simulink library "vmc"  (R2021b)
settings: Solver=VariableStepAuto  StartTime=0.0  StopTime=10.0  RelTol=1e-3
undefined symbols (not defined in the file or in its folder): AVMC_ACCDeltaTqIGain_X_kph, AVMC_ACCDeltaTqIGain_Y_mps2, AVMC_ACCDeltaTqPGain_X_kph, AVMC_ACCDeltaTqPGain_Y_kph, AVMC_ACCLongSteadyCtrl_X_kph, AVMC_AggressJerkPCT4AT_X_kph, AVMC_AggressJerkPCT_X_kph, AVMC_AggressLimitPCT4AT_X_kph, AVMC_AggressLimitPCT_X_kph, AVMC_CCLongSteadyCtrl_X_kph, AVMC_DISCDeltaTqIGain_X_kph, AVMC_DISCDeltaTqIGain_Y_mps2, AVMC_DISCDeltaTqPGain_X_kph, AVMC_DISCDeltaTqPGain_Y_kph, AVMC_DISCTrunAccJerk_X_s, AVMC_DISCTrunAccLimit_X_s, AVMC_ESCRegenOut_X_kph, AVMC_ESCRegenOut_Y_Deg, AVMC_ESCRegenOutEnSpd_X_Deg, AVMC_ISOAccLimit_X_mps, AVMC_ISODecLimit_X_mps, AVMC_ISOJerk_X_mps, AVMC_LatESCRegenOut_X_kph, AVMC_LatESCRegenOut_Y_Deg, AVMC_LongAccDeadZone_X_kph, AVMC_LongAccFiltTsforP2_X_Gps, AVMC_MCPresBaseTq_X_bar, AVMC_MSALongSteadyCtrl_X_kph, AVMC_MSAPedalOvrd2_X_kph, AVMC_MSAPedalOvrd_X_kph, AVMC_MSASpdBand_X_kph, AVMC_MSATqDownEndTq_X_kph, AVMC_MSATqDownTime_X_kph, AVMC_RDCDetectTime_X_kph, AVMC_RDCDetectTime_Y_pct, AVMC_RDCEnSlideRate_X_Deg, AVMC_RearWhlTqRatio_X_Nm, AVMC_RearWhlTqRatio_Y_gps, AVMC_RearWhlTqSlipGain_X_rat, AVMC_RearWhlTqSlipGain_Y_kph, AVMC_SoftJerkPCT_X_kph, AVMC_SoftLimitPCT_X_kph, AVMC_StESCYaw_X_kph, AVMC_StESCYaw_Y_Deg, AVMC_StESCYawCom_X_kph, AVMC_StESCYawCom_Y_Gps, AVMC_TMSpdBaseTq_X_rpm, AVMC_VehHoldBDecMap_X_kph, AVMC_VehHoldDecCtrlTime_X_kph, AVMC_VehHoldMCPPass_X_deg, C_TASK_10MS_S, C_TASK_5MS_S, DEG2RAD, Discrete, ENUM_ACCAVAIL_AVAILABLE, ENUM_ACCCTRLALLOW_ALLOW, ENUM_ADASACCSTA_ACTIVE, ENUM_ADASACCSTA_OVERRIDE, ENUM_ADASACCSTA_SHUTOFF, ENUM_ADASAEBREQ_NOREQUEST ... (+361)
libraries: hcu_lib x63, simulink x60, simulink_extras x3, ctrlSharedLib x3, $bdroot x2
(part 7 of 15)

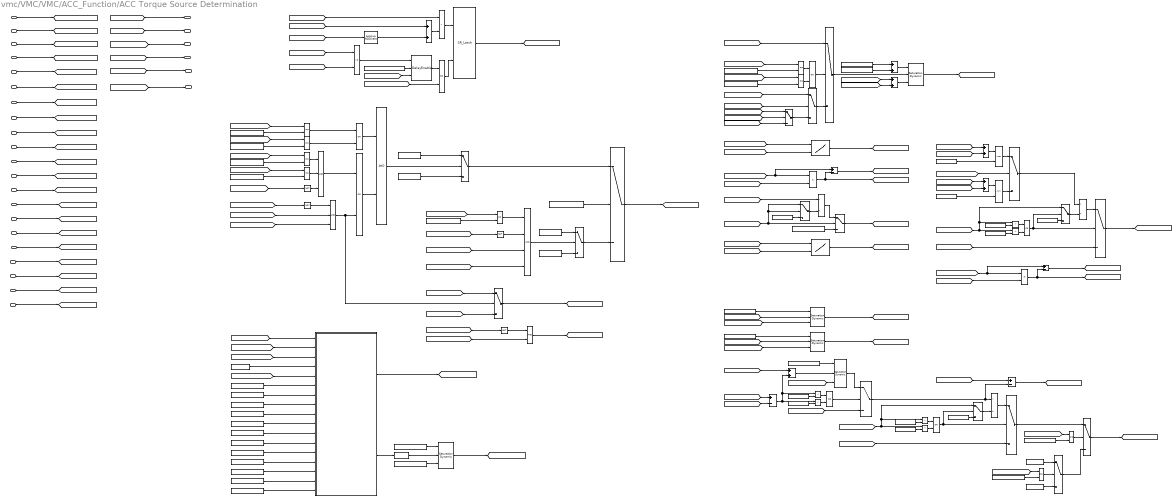
== system vmc/VMC/VMC/ACC_Function/ACC Torque Source Determination ==
  note: TRUE
  VTQD_DriverWhlTqDem_Nm : Inport
  VVMC_ADASWhlTqCal_Nm : Inport  Port=2
  VVMC_FeatArbitrFinal_enum : Inport  Port=3
  VTQD_LowIdleAccPedal_flg : Inport  Port=4
  VINP_ACCObjDist_m : Inport  Port=5
  VINP_TimeGapLevel_enum : Inport  Port=6
  VVMC_FeatArbitrSta_enum : Inport  Port=7
  VINP_RegenMode_enum : Inport  Port=8
  VVMC_ADASActive_flg : Inport  Port=9
  task_time_s : Inport  Port=10
  VINP_LongAccel_Gps : Inport  Port=11
  VINP_VehSpeed_kph : Inport  Port=12
  VVMC_FrRrSlipSpd_kph : Inport  Port=13
  VVMC_CruzWhlTqReq_Nm : Inport  Port=14
  VVMC_CruzActive_flg : Inport  Port=15
  VVMC_MSAWhlTqReq_Nm : Inport  Port=16
  VVMC_MSAActive_flg : Inport  Port=17
  VTQD_RrEDUAvailBrkRgnTq_Nm : Inport  Port=18
  VTQD_FrEDUAvailBrkRgnTq_Nm : Inport  Port=19
  VPMM_DrivetrainSelect_enum : Inport  Port=20
  VINP_ACCObjRelSpd_mps : Inport  Port=21
  AND : Logic  AllPortsSameDT=off  OutDataTypeStr=boolean
  AND1 : Logic  Inputs=4  AllPortsSameDT=off  OutDataTypeStr=boolean
  AND2 : Logic  Operator=OR  AllPortsSameDT=off  OutDataTypeStr=boolean
  AND3 : Logic  Operator=OR  AllPortsSameDT=off  OutDataTypeStr=boolean
  AND4 : Logic  Operator=OR  AllPortsSameDT=off  OutDataTypeStr=boolean
  Add{,2..3,9..11} (6 alike) : Sum
  Add{1,4..6} (4 alike) : Sum  Inputs=+-
  Cast To Single : DataTypeConversion  OutDataTypeStr=single
  Constant : Constant  Value=KVMC_ACCPedalOvrdSWC_flg
  Constant1 : Constant  Value=FALSE
  Constant10 : Constant  Value=ENUM_TIMEGAPLEVEL_LEVEL1
  Constant11 : Constant  Value=ENUM_TIMEGAPLEVEL_LEVEL2
  Constant12 : Constant  Value=ENUM_TIMEGAPLEVEL_LEVEL3
  Constant13 : Constant  Value=ENUM_TIMEGAPLEVEL_LEVEL4
  Constant14 : Constant  Value=KVMC_TimeGapBandLv2_s
  Constant15 : Constant  Value=KVMC_TimeGapBandLv3_s
  Constant16 : Constant  Value=KVMC_TimeGapBandLv4_s
  Constant17 : Constant  Value=TRUE
  Constant18 : Constant  Value=FALSE
  Constant{19,24..26,39,41..46,48} (12 alike) : Constant  Value=ZERO_FLOAT
  Constant2 : Constant  Value=ENUM_FEATARBITRSTA_DISC
  Constant20 : Constant  Value=FALSE
  Constant21 : Constant  Value=ENUM_FEATARBITRSTA_ACC
  Constant22 : Constant  Value=TRUE
  Constant23 : Constant  Value=KVMC_ACCPedalOvrdRestTime_s
  Constant{27..28,37,40} (4 alike) : Constant  Value=ONE_FLOAT
  Constant29 : Constant  Value=ENUM_FEATARBITRSTA_ACC
  Constant3 : Constant  Value=TRUE
  Constant30 : Constant  Value=ENUM_FEATARBITRSTA_DISC
  Constant31 : Constant  Value=KTQD_RrUppTheldTrq_Nm
  Constant32 : Constant  Value=ENUM_DRIVETRAIN_AWD  VectorParams1D=off  SampleTime=-1
  Constant33 : Constant  Value=KTQD_RrUppTheldTrq_Nm
  Constant34 : Constant  Value=KTQD_RrUppTheldTrq_Nm
  Constant35 : Constant  Value=KTQD_FrUppTheldTrq_Nm
  Constant36 : Constant  Value=KTQD_FrUppTheldTrq_Nm
  Constant38 : Constant  Value=ENUM_DRIVETRAIN_RWD  VectorParams1D=off  SampleTime=-1
  Constant4 : Constant  Value=ENUM_FEATARBITRSTA_ACC
  Constant47 : Constant  Value=KVMC_TimeGapMax_s
  Constant5 : Constant  Value=ENUM_FEATARBITRSTA_DISC
  Constant6 : Constant  Value=ENUM_FEATARBITRSTA_ACCDISC
  Constant7 : Constant  Value=KVMC_TimeGapMax_s
  Constant8 : Constant  Value=KPH2MPS
  Constant9 : Constant  Value=KVMC_TimeGapBandLv1_s
  DelayEnable : hcu_lib/Basic_Blocks/DelayEnable
  Direct Lookup Table (n-D)1 : LookupNDDirect  NumberOfTableDimensions=1  Table=MVMC_ACCPedalOvrdTqHys_Y_Nm
  Divide : Product  Inputs=**
  Divide1 : Product  Inputs=*/
  Divide2 : Product  Inputs=*/
  Divide3 : Product  Inputs=**
  Divide4 : Product  Inputs=*/
  Equal1 : RelationalOperator  Operator===  OutDataTypeStr=boolean  RndMeth=Simplest
  Equal3 : RelationalOperator  Operator===  OutDataTypeStr=boolean  RndMeth=Simplest
  Logical Operator : Logic  Operator=OR  AllPortsSameDT=off  OutDataTypeStr=boolean
  Logical Operator1 : Logic  Inputs=3  AllPortsSameDT=off  OutDataTypeStr=boolean
  Logical Operator2 : Logic  Operator=OR  AllPortsSameDT=off  OutDataTypeStr=boolean
  Logical Operator3 : Logic  Inputs=3  AllPortsSameDT=off  OutDataTypeStr=boolean
  Logical Operator4 : Logic  AllPortsSameDT=off  OutDataTypeStr=boolean
  Logical Operator5 : Logic  Operator=OR  AllPortsSameDT=off  OutDataTypeStr=boolean
  MMAP_RearWhlTqSlipGain_Z_Nm : Lookup_n-D  BreakpointsForDimension1=AVMC_RearWhlTqSlipGain_Y_kph  BreakpointsForDimension2=AVMC_RearWhlTqSlipGain_X_rat  Table=MVMC_RearWhlTqSlipGain_Z_Nm  InternalRulePriority=Speed  RndMeth=Simplest  InputSameDT=on
      settings: InputPortMap=u0,u1
  MVMC_RearWhlTqRatio_Z_rat : Lookup_n-D  BreakpointsForDimension1=AVMC_RearWhlTqRatio_Y_gps  BreakpointsForDimension2=AVMC_RearWhlTqRatio_X_Nm  Table=MVMC_RearWhlTqRatio_Z_rat  InternalRulePriority=Speed  RndMeth=Simplest  InputSameDT=on
      settings: InputPortMap=u0,u1
  Max : MinMax  Function=max  Inputs=2
  Max1 : MinMax  Inputs=2
  NOT{,1..3} (4 alike) : Logic  Operator=NOT  AllPortsSameDT=off  OutDataTypeStr=boolean
  OR1 : Logic  Operator=OR  AllPortsSameDT=off  OutDataTypeStr=boolean
  Relational Operator{,7,11,13} (4 alike) : RelationalOperator  Operator=>  OutDataTypeStr=boolean  RndMeth=Simplest
  Relational Operator{1..6,9} (7 alike) : RelationalOperator  Operator===  OutDataTypeStr=boolean  RndMeth=Simplest
  Relational Operator10 : RelationalOperator  Operator=<  OutDataTypeStr=boolean  RndMeth=Simplest
  Relational Operator12 : RelationalOperator  Operator=<  OutDataTypeStr=boolean  RndMeth=Simplest
  Relational Operator14 : RelationalOperator  Operator=<  OutDataTypeStr=boolean  RndMeth=Simplest
  Relational Operator8 : RelationalOperator  Operator=<=  OutDataTypeStr=boolean  RndMeth=Simplest
  SR_Latch : hcu_lib/Basic_Blocks/SR_Latch
  Saturation Dynamic{,1..4} (5 alike) : simulink/Discontinuities/Saturation Dynamic  OutMin=[]  OutMax=[]  OutDataTypeStr=Inherit: Same as second input  OutDataType=fixdt(1, 16)  OutScaling=2^-10  DoSatur=off
  Switch{,4..7,9..10} (7 alike) : Switch  Criteria=u2 > Threshold
  Switch{1,3,8,11,13} (5 alike) : Switch  Criteria=u2 ~= 0
  Switch2 : Switch
  TimeGapJudgement : Stateflow chart  TreatAsAtomicUnit=on
  u2 > 0 : Switch  Criteria=u2 > Threshold
  u2 > 0 (1) : Switch  Criteria=u2 > Threshold
  u2 > 0 (2) : Switch  Criteria=u2 > Threshold
  u2 > 0 (3) : Switch  Criteria=u2 > Threshold
  VVMC_ACCPedalOvrd_flg : Outport
  VVMC_ADASWhlTqReq_Nm : Outport  Port=2
  VVMC_TimeGapCalcu_s : Outport  Port=3
  VVMC_AccPedalOvrdDISC_flg : Outport  Port=4
  VVMC_RearTqRatio_rat : Outport  Port=5
  VVMC_TimeGapJudge_flag : Outport  Port=6
  wires:
  [VVMC_ACCPedalTqEnOvrd_flg] -> Logical Operator1/2
  [VVMC_ADASActive_flg] -> AND1/4
  [VVMC_ACCPedalTqEnOvrd_flg] -> AND1/3
  [VVMC_ADASWhlTqCal_Nm] -> Relational Operator8/2
  [VTQD_DriverWhlTqDem_Nm] -> Relational Operator7/1
  Relational Operator8/1 -> DelayEnable/1
  SR_Latch/1 -> [VVMC_ACCPedalTqEnOvrd_flg]  "VVMC_ACCPedalTqEnOvrd_flg"
  Direct Lookup Table (n-D)1/1 -> Add/2  "VVMC_ACCPedalOvrdTqHys_Nm"
  [VTQD_DriverWhlTqDem_Nm] -> Relational Operator8/1
  Relational Operator7/1 -> SR_Latch/1
  Add/1 -> Relational Operator7/2
  [VVMC_ADASWhlTqCal_Nm] -> Add/1
  [VINP_RegenMode_enum] -> Direct Lookup Table (n-D)1/1
  VVMC_ADASActive_flg/1 -> [VVMC_ADASActive_flg]
  VINP_RegenMode_enum/1 -> [VINP_RegenMode_enum]
  Saturation Dynamic2/1 -> [VVMC_TimeGapCalcu_s]  "VVMC_TimeGapCalcu_s"
  Constant/1 -> u2 > 0 (3)/2
  u2 > 0/1 -> u2 > 0 (3)/1
  u2 > 0 (2)/1 -> u2 > 0 (3)/3
  [VVMC_FeatArbitrFinal_enum] -> Relational Operator6/1
  Constant21/1 -> Relational Operator6/2
  Constant22/1 -> u2 > 0 (2)/1
  Constant20/1 -> u2 > 0 (2)/3
  NOT2/1 -> AND1/2
  [VTQD_LowIdleAccPedal_flg] -> NOT2/1
  AND1/1 -> u2 > 0 (2)/2
  Relational Operator6/1 -> AND1/1
  [VVMC_TimeGapCalcu_s] -> VVMC_TimeGapCalcu_s/1
  TimeGapJudgement/2(VVMC_TimeGapCalcu_s) -> Cast To Single/1
  Constant7/1 -> TimeGapJudgement/17(KVMC_TimeGapMax_s)
  Constant6/1 -> Relational Operator4/2
  [VVMC_FeatArbitrSta_enum] -> Relational Operator4/1
  Relational Operator4/1 -> Logical Operator3/1
  VVMC_FeatArbitrSta_enum/1 -> [VVMC_FeatArbitrSta_enum]
  Constant19/1 -> TimeGapJudgement/16(ZERO_FLOAT)
  Constant18/1 -> TimeGapJudgement/15(FALSE)
  Constant17/1 -> TimeGapJudgement/14(TRUE)
  Constant16/1 -> TimeGapJudgement/13(KVMC_TimeGapBandLv4_s)
  Constant13/1 -> TimeGapJudgement/12(ENUM_TIMEGAPLEVEL_LEVEL4)
  Constant15/1 -> TimeGapJudgement/11(KVMC_TimeGapBandLv3_s)
  Constant12/1 -> TimeGapJudgement/10(ENUM_TIMEGAPLEVEL_LEVEL3)
  Constant14/1 -> TimeGapJudgement/9(KVMC_TimeGapBandLv2_s)
  Constant11/1 -> TimeGapJudgement/8(ENUM_TIMEGAPLEVEL_LEVEL2)
  Constant9/1 -> TimeGapJudgement/7(KVMC_TimeGapBandLv1_s)
  Constant10/1 -> TimeGapJudgement/6(ENUM_TIMEGAPLEVEL_LEVEL1)
  [VVMC_TimeGapJudge_flag] -> NOT1/1
  NOT1/1 -> Logical Operator3/3
  Relational Operator1/1 -> Logical Operator3/2
  TimeGapJudgement/1(VVMC_TimeGapJudge_flag) -> [VVMC_TimeGapJudge_flag]  "VVMC_TimeGapJudge_flag"
  [VINP_ACCObjDist_m] -> TimeGapJudgement/2(VINP_ACCObjDist_m)
  [VINP_VehSpeed_kph] -> TimeGapJudgement/3(VINP_VehSpeed_kph)
  Constant8/1 -> TimeGapJudgement/4(KPH2MPS)
  [VINP_TimeGapLevel_enum] -> TimeGapJudgement/5(VINP_TimeGapLevel_enum)
  VINP_TimeGapLevel_enum/1 -> [VINP_TimeGapLevel_enum]
  VINP_ACCObjDist_m/1 -> [VINP_ACCObjDist_m]
  Logical Operator2/1 -> AND/1
  Relational Operator3/1 -> Logical Operator2/2
  Constant5/1 -> Relational Operator3/2
  [VVMC_FeatArbitrFinal_enum] -> Relational Operator3/1
  Logical Operator/1 -> AND/2
  Logical Operator3/1 -> Logical Operator/1
  [VVMC_FeatArbitrFinal_enum] -> Relational Operator1/1
  Constant2/1 -> Relational Operator1/2
  Constant4/1 -> Relational Operator2/2
  [VVMC_FeatArbitrFinal_enum] -> Relational Operator2/1
  VTQD_DriverWhlTqDem_Nm/1 -> [VTQD_DriverWhlTqDem_Nm]
  VVMC_ADASWhlTqCal_Nm/1 -> [VVMC_ADASWhlTqCal_Nm]
  [VVMC_ACCPedalOvrd_flg] -> VVMC_ACCPedalOvrd_flg/1
  [VVMC_ADASWhlTqReq_Nm] -> VVMC_ADASWhlTqReq_Nm/1
  u2 > 0 (1)/1 -> [VVMC_ADASWhlTqReq_Nm]  "VVMC_ADASWhlTqReq_Nm"
  [VVMC_ADASWhlTqCal_Nm] -> u2 > 0 (1)/3
  [VTQD_DriverWhlTqDem_Nm] -> u2 > 0 (1)/1
  Constant1/1 -> u2 > 0/3
  Constant3/1 -> u2 > 0/1
  u2 > 0 (3)/1 -> [VVMC_ACCPedalOvrd_flg]  "VVMC_ACCPedalOvrd_flg"
  AND/1 -> u2 > 0/2
  Relational Operator2/1 -> Logical Operator2/1
  VVMC_FeatArbitrFinal_enum/1 -> [VVMC_FeatArbitrFinal_enum]
  VTQD_LowIdleAccPedal_flg/1 -> [VTQD_LowIdleAccPedal_flg]
  NOT/1 -> Logical Operator1/1
  [VTQD_LowIdleAccPedal_flg] -> NOT/1
  [VVMC_AccPedalOvrdDISC_flg] -> VVMC_AccPedalOvrdDISC_flg/1
  Logical Operator4/1 -> [VVMC_AccPedalOvrdDISC_flg]  "VVMC_AccPedalOvrdDISC_flg"
  NOT3/1 -> Logical Operator4/1
  [VVMC_ACCPedalTqEnOvrd_flg] -> Logical Operator4/2
  [VTQD_LowIdleAccPedal_flg] -> NOT3/1
  [task_time_s] -> DelayEnable/3
  DelayEnable/1 -> OR1/1
  Constant23/1 -> DelayEnable/2
  [VTQD_LowIdleAccPedal_flg] -> OR1/2
  OR1/1 -> SR_Latch/2
  task_time_s/1 -> [task_time_s]
  [VVMC_VMCWhlTq4RatioCalcu_Nm] -> MVMC_RearWhlTqRatio_Z_rat/2
  VINP_LongAccel_Gps/1 -> [VINP_LongAccel_Gps]
  [VINP_LongAccel_Gps] -> MVMC_RearWhlTqRatio_Z_rat/1
  MVMC_RearWhlTqRatio_Z_rat/1 -> [VVMC_RearTqRatioBfrSlip_rat]  "VVMC_RearTqRatioBfrSlip_rat"
  [VVMC_RearTqRatio_rat] -> VVMC_RearTqRatio_rat/1
  VINP_VehSpeed_kph/1 -> [VINP_VehSpeed_kph]
  VVMC_FrRrSlipSpd_kph/1 -> [VVMC_FrRrSlipSpd_kph]
  [VVMC_VMCWhlTq4RatioCalcu_Nm] -> Divide/1, Add1/1
  [VVMC_RearTqRatioBfrSlip_rat] -> Divide/2
  Divide/1 -> [VVMC_ADASRrWhlTqBfrSlip_Nm], Add1/2  "VVMC_ADASRrWhlTqBfrSlip_Nm"
  Add1/1 -> [VVMC_ADASFrWhlTqBfrSlip_Nm]  "VVMC_ADASFrWhlTqBfrSlip_Nm"
  [VINP_VehSpeed_kph] -> Switch/2, Switch4/2, Switch4/1
  Constant24/1 -> Switch/3
  Divide1/1 -> Switch/1
  [VVMC_FrRrSlipSpd_kph] -> Divide1/1
  Switch/1 -> [VVMC_FrRrSlipRate_rat]  "VVMC_FrRrSlipRate_rat"
  [VVMC_FrRrSlipRate_rat] -> MMAP_RearWhlTqSlipGain_Z_Nm/2
  [VINP_VehSpeed_kph] -> MMAP_RearWhlTqSlipGain_Z_Nm/1
  MMAP_RearWhlTqSlipGain_Z_Nm/1 -> [VVMC_RearWhlTqSlipGain_Nm]  "VVMC_RearWhlTqSlipGain_Nm"
  [VVMC_ADASRrWhlTqBfrSlip_Nm] -> Add2/1
  [VVMC_RearWhlTqSlipGain_Nm] -> Add2/2
  [VVMC_RearTqRatioBfrSlip_rat] -> Switch1/3
  Add2/1 -> Max/1
  [VVMC_VMCWhlTq4RatioCalcu_Nm] -> Switch2/2
  Switch1/1 -> [VVMC_RearTqRatioAftSlip_rat]  "VVMC_RearTqRatioAftSlip_rat"
  Max/1 -> Switch2/1
  Constant25/1 -> Max/2
  Constant26/1 -> Max1/2
  Add3/1 -> Max1/1
  [VVMC_RearWhlTqSlipGain_Nm] -> Add3/2
  [VVMC_ADASRrWhlTqBfrSlip_Nm] -> Add3/1
  Max1/1 -> Switch2/3
  Switch2/1 -> Divide2/1
  Divide2/1 -> Switch1/1
  Constant27/1 -> Switch3/3
  Switch3/1 -> Divide2/2
  Constant28/1 -> Switch4/3
  Switch4/1 -> Divide1/2
  [VVMC_ADASActive_flg] -> Logical Operator1/3
  Relational Operator5/1 -> Logical Operator5/1
  Relational Operator9/1 -> Logical Operator5/2
  [VVMC_FeatArbitrFinal_enum] -> Relational Operator5/1
  Constant30/1 -> Relational Operator9/2
  [VVMC_FeatArbitrFinal_enum] -> Relational Operator9/1
  Constant29/1 -> Relational Operator5/2
  Logical Operator5/1 -> Switch5/2
  [VTQD_DriverWhlTqDem_Nm] -> Switch7/3
  [VVMC_ADASWhlTqReq_Nm] -> Switch5/1
  Saturation Dynamic4/1 -> [VVMC_VMCWhlTq4RatioCalcu_Nm]  "VVMC_VMCWhlTq4RatioCalcu_Nm"
  VVMC_MSAActive_flg/1 -> [VVMC_MSAActive_flg]
  VVMC_MSAWhlTqReq_Nm/1 -> [VVMC_MSAWhlTqReq_Nm]
  VVMC_CruzWhlTqReq_Nm/1 -> [VVMC_CruzWhlTqReq_Nm]
  VVMC_CruzActive_flg/1 -> [VVMC_CruzActive_flg]
  [VVMC_CruzActive_flg] -> Switch6/2
  [VVMC_CruzWhlTqReq_Nm] -> Switch6/1
  Switch6/1 -> Switch5/3
  [VVMC_MSAActive_flg] -> Switch7/2
  [VVMC_MSAWhlTqReq_Nm] -> Switch7/1
  Switch7/1 -> Switch6/3
  Add4/1 -> [VVMC_ADASFrWhlTqAftSlip_Nm]  "VVMC_ADASFrWhlTqAftSlip_Nm"
  Divide3/1 -> Add4/2, [VVMC_ADASRrWhlTqAftSlip_Nm]  "VVMC_ADASRrWhlTqAftSlip_Nm"
  [VVMC_RearTqRatioAftSlip_rat] -> Divide3/2
  [VVMC_VMCWhlTq4RatioCalcu_Nm] -> Add4/1, Divide3/1
  VTQD_FrEDUAvailBrkRgnTq_Nm/1 -> [VTQD_FrEDUAvailBrkRgnTq_Nm]
  VTQD_RrEDUAvailBrkRgnTq_Nm/1 -> [VTQD_RrEDUAvailBrkRgnTq_Nm]
  [VVMC_ADASFrWhlTqAftSlip_Nm] -> Saturation Dynamic/2
  Constant35/1 -> Saturation Dynamic/1
  [VTQD_FrEDUAvailBrkRgnTq_Nm] -> Saturation Dynamic/3
  Constant31/1 -> Saturation Dynamic1/1
  [VVMC_ADASRrWhlTqAftSlip_Nm] -> Saturation Dynamic1/2
  [VTQD_RrEDUAvailBrkRgnTq_Nm] -> Saturation Dynamic1/3
  Saturation Dynamic/1 -> [VVMC_ADASFrWhlTqAftLim_Nm]  "VVMC_ADASFrWhlTqAftLim_Nm"
  Saturation Dynamic1/1 -> [VVMC_ADASRrWhlTqAftLim_Nm]  "VVMC_ADASRrWhlTqAftLim_Nm"
  [VVMC_ADASFrWhlTqAftSlip_Nm] -> Add5/1
  [VVMC_ADASFrWhlTqAftLim_Nm] -> Add5/2
  [VVMC_ADASRrWhlTqAftLim_Nm] -> Switch8/3
  Saturation Dynamic3/1 -> Switch8/1
  [VVMC_ADASRrWhlTqAftLim_Nm] -> Add9/1
  Constant33/1 -> Saturation Dynamic3/1
  [VTQD_RrEDUAvailBrkRgnTq_Nm] -> Saturation Dynamic3/3
  Add9/1 -> Saturation Dynamic3/2
  Switch13/1 -> Divide4/2
  Constant37/1 -> Switch13/3
  Divide4/1 -> Switch11/1
  Switch8/1 -> Add6/2, Divide4/1  "VVMC_ADASRrWhlTq_Nm"
  Switch9/1 -> [VVMC_RearTqRatio_rat]  "VVMC_RearTqRatio_rat"
  [VVMC_RearTqRatioBfrSlip_rat] -> Switch11/3
  [VTQD_RrEDUAvailBrkRgnTq_Nm] -> Add11/2
  Constant34/1 -> Add10/2
  [VTQD_FrEDUAvailBrkRgnTq_Nm] -> Add11/1
  Constant36/1 -> Add10/1
  Add10/1 -> Saturation Dynamic4/1
  Add11/1 -> Saturation Dynamic4/3
  Switch5/1 -> Saturation Dynamic4/2
  [VVMC_VMCWhlTq4RatioCalcu_Nm] -> Add6/1
  Add6/1 -> [VVMC_ADASFrWhlTq_Nm]  "VVMC_ADASFrWhlTq_Nm"
  VPMM_DrivetrainSelect_enum/1 -> [VPMM_DrivetrainSelect_enum]
  [VPMM_DrivetrainSelect_enum] -> Equal3/1
  Constant32/1 -> Equal3/2
  Switch11/1 -> Switch9/1
  Equal3/1 -> Switch9/2
  Constant38/1 -> Equal1/2
  [VPMM_DrivetrainSelect_enum] -> Equal1/1
  Equal1/1 -> Switch10/2
  Switch10/1 -> Switch9/3
  Constant39/1 -> Switch10/3
  Constant40/1 -> Switch10/1
  Constant42/1 -> Relational Operator10/2
  Relational Operator/1 -> AND2/1
  Relational Operator10/1 -> AND2/2
  Constant41/1 -> Relational Operator/2
  [VVMC_VMCWhlTq4RatioCalcu_Nm] -> Relational Operator10/1, Switch3/1, Relational Operator/1
  AND2/1 -> Switch3/2, Switch1/2
  Constant44/1 -> Relational Operator12/2
  Relational Operator11/1 -> AND3/1
  Relational Operator12/1 -> AND3/2
  Constant43/1 -> Relational Operator11/2
  Add5/1 -> Relational Operator11/1, Add9/2, Relational Operator12/1
  AND3/1 -> Switch8/2
  Constant46/1 -> Relational Operator14/2
  Relational Operator13/1 -> AND4/1
  Relational Operator14/1 -> AND4/2
  Constant45/1 -> Relational Operator13/2
  [VVMC_VMCWhlTq4RatioCalcu_Nm] -> Relational Operator14/1, Switch13/1, Relational Operator13/1
  AND4/1 -> Switch13/2, Switch11/2
  VINP_ACCObjRelSpd_mps/1 -> [VINP_ACCObjRelSpd_mps]
  [VINP_ACCObjRelSpd_mps] -> TimeGapJudgement/1(VINP_ACCObjRelSpd_mps)
  Cast To Single/1 -> Saturation Dynamic2/2
  Constant47/1 -> Saturation Dynamic2/1
  Constant48/1 -> Saturation Dynamic2/3
  Logical Operator1/1 -> u2 > 0 (1)/2, Logical Operator/2
  [VVMC_TimeGapJudge_flag] -> VVMC_TimeGapJudge_flag/1

== system vmc/VMC/VMC/ACC_Function/Hand Shaking ==
  VVMC_FeatArbitrFinal_enum : Inport
  VVMC_ACCCtrlAllow_flg : Inport  Port=2
  Constant1 : Constant  Value=TRUE
  Constant2 : Constant  Value=ENUM_FEATARBITRSTA_DISC
  Constant3 : Constant  Value=FALSE
  Constant4 : Constant  Value=ENUM_FEATARBITRSTA_ACC
  Constant5 : Constant  Value=TRUE
  Constant6 : Constant  Value=FALSE
  Logical Operator : Logic  AllPortsSameDT=off  OutDataTypeStr=boolean
  Logical Operator1 : Logic  Operator=OR  AllPortsSameDT=off  OutDataTypeStr=boolean
  Relational Operator1 : RelationalOperator  Operator===  OutDataTypeStr=boolean  RndMeth=Simplest
  Relational Operator2 : RelationalOperator  Operator===  OutDataTypeStr=boolean  RndMeth=Simplest
  Switch : Switch  Criteria=u2 > Threshold
  u2>0 : Switch  Criteria=u2 > Threshold
  VVMC_ACCCtrlAvail_flg : Outport
  VVMC_ADASActive_flg : Outport  Port=2
  wires:
  Logical Operator1/1 -> Logical Operator/1
  Relational Operator2/1 -> Logical Operator1/1
  Constant4/1 -> Relational Operator2/2
  [VVMC_FeatArbitrFinal_enum] -> Relational Operator2/1
  [VVMC_ACCCtrlAvail_flg] -> VVMC_ACCCtrlAvail_flg/1
  VVMC_FeatArbitrFinal_enum/1 -> [VVMC_FeatArbitrFinal_enum]
  [VVMC_FeatArbitrFinal_enum] -> Relational Operator1/1
  Constant2/1 -> Relational Operator1/2
  [VVMC_ADASActive_flg] -> VVMC_ADASActive_flg/1
  [VVMC_ACCCtrlAllow_flg] -> Logical Operator/2, Switch/2
  Switch/1 -> [VVMC_ACCCtrlAvail_flg]  "VVMC_ACCCtrlAvail_flg"
  Constant6/1 -> Switch/3
  Constant5/1 -> Switch/1
  VVMC_ACCCtrlAllow_flg/1 -> [VVMC_ACCCtrlAllow_flg]
  Relational Operator1/1 -> Logical Operator1/2
  Logical Operator/1 -> u2>0/2
  Constant1/1 -> u2>0/1
  u2>0/1 -> [VVMC_ADASActive_flg]  "VVMC_ADASActive_flg"
  Constant3/1 -> u2>0/3

== system vmc/VMC/VMC/APS function/Command Determination ==
  VVMC_APSActive_flg : Inport
  VINP_APSStaSys_enum : Inport  Port=2
  VINP_APSShiftPosnReq_enum : Inport  Port=3
  VINP_APSSpeedCMD_kph : Inport  Port=4
  AND : Logic  AllPortsSameDT=off  OutDataTypeStr=boolean
  Constant : Constant  Value=ENUM_APSSYSTEMSTA_ACTIVE
  Constant1 : Constant  Value=ENUM_APSSYSTEMSTA_REMOTEACTIVE
  Constant2 : Constant  Value=ZERO_FLOAT
  Constant3 : Constant  Value=ENUM_APSSHIFTPOSNREQ_PARK
  Equal : RelationalOperator  Operator===  OutDataTypeStr=boolean  RndMeth=Simplest
  Equal1 : RelationalOperator  Operator===  OutDataTypeStr=boolean  RndMeth=Simplest
  OR : Logic  Operator=OR  AllPortsSameDT=off  OutDataTypeStr=boolean
  Switch : Switch  Criteria=u2 > Threshold
  Switch1 : Switch  Criteria=u2 > Threshold
  VVMC_APSSpeedCMD_kph : Outport
  VVMC_APSShiftPosnReq_enum : Outport  Port=2
  wires:
  [VVMC_APSEnCMD_flg] -> Switch1/2
  [VINP_APSShiftPosnReq_enum] -> Switch1/1
  Constant3/1 -> Switch1/3
  Switch1/1 -> VVMC_APSShiftPosnReq_enum/1  "VVMC_APSShiftPosnReq_enum"
  Switch/1 -> VVMC_APSSpeedCMD_kph/1  "VVMC_APSSpeedCMD_kph"
  Constant2/1 -> Switch/3
  [VINP_APSSpeedCMD_kph] -> Switch/1
  [VVMC_APSEnCMD_flg] -> Switch/2
  AND/1 -> [VVMC_APSEnCMD_flg]  "VVMC_APSEnCMD_flg"
  OR/1 -> AND/2
  [VVMC_APSActive_flg] -> AND/1
  Equal1/1 -> OR/2
  Equal/1 -> OR/1
  [VINP_APSStaSys_enum] -> Equal1/1
  Constant1/1 -> Equal1/2
  Constant/1 -> Equal/2
  [VINP_APSStaSys_enum] -> Equal/1
  VINP_APSSpeedCMD_kph/1 -> [VINP_APSSpeedCMD_kph]
  VINP_APSShiftPosnReq_enum/1 -> [VINP_APSShiftPosnReq_enum]
  VINP_APSStaSys_enum/1 -> [VINP_APSStaSys_enum]
  VVMC_APSActive_flg/1 -> [VVMC_APSActive_flg]

== system vmc/VMC/VMC/APS function/Hand Shake ==
  task_time_s : Inport
  VTQD_ExternalTqAllow_flg : Inport  Port=2
  VTQD_ExtShiftAllow_flg : Inport  Port=3
  VINP_APSVMCReqA_flg : Inport  Port=4
  VINP_APSStaSys_enum : Inport  Port=5
  VTQD_ExtDoorAllow_flg : Inport  Port=6
  AND : Logic  Inputs=3  AllPortsSameDT=off  OutDataTypeStr=boolean
  AND1 : Logic  Inputs=3  AllPortsSameDT=off  OutDataTypeStr=boolean
  Constant : Constant  Value=KVMC_ExternalTqAllowTime_s
  Constant1 : Constant  Value=KVMC_ExternalShiftAllowTime_s
  Constant2 : Constant  Value=ENUM_APSSYSTEMSTA_ACTIVE
  Constant3 : Constant  Value=ENUM_APSSYSTEMSTA_REMOTEACTIVE
  Constant4 : Constant  Value=KVMC_ExternalDoorAllowTime_s
  DelayEnable : hcu_lib/Basic_Blocks/DelayEnable
  DelayEnable1 : hcu_lib/Basic_Blocks/DelayEnable
  DelayEnable2 : hcu_lib/Basic_Blocks/DelayEnable
  Equal : RelationalOperator  Operator===  OutDataTypeStr=boolean  RndMeth=Simplest
  Equal1 : RelationalOperator  Operator===  OutDataTypeStr=boolean  RndMeth=Simplest
  OR : Logic  Operator=OR  AllPortsSameDT=off  OutDataTypeStr=boolean
  VVMC_APSCtrlAvail_flg : Outport
  VVMC_APSActive_flg : Outport  Port=2
  wires:
  VINP_APSVMCReqA_flg/1 -> [VINP_APSVMCReqA_flg]
  AND/1 -> VVMC_APSCtrlAvail_flg/1, [VVMC_APSCtrlAvail_flg]  "VVMC_APSCtrlAvail_flg"
  [VVMC_APSShiftCtrlAllow_flg] -> AND/2
  [VVMC_APSTqCtrlAllow_flg] -> AND/1
  VTQD_ExtShiftAllow_flg/1 -> [VTQD_ExtShiftAllow_flg]
  [task_time_s] -> DelayEnable1/3
  Constant1/1 -> DelayEnable1/2
  DelayEnable1/1 -> [VVMC_APSShiftCtrlAllow_flg]  "VVMC_APSShiftCtrlAllow_flg"
  [VTQD_ExtShiftAllow_flg] -> DelayEnable1/1
  [VTQD_ExternalTqAllow_flg] -> DelayEnable/1
  VTQD_ExternalTqAllow_flg/1 -> [VTQD_ExternalTqAllow_flg]
  task_time_s/1 -> [task_time_s]
  DelayEnable/1 -> [VVMC_APSTqCtrlAllow_flg]  "VVMC_APSTqCtrlAllow_flg"
  Constant/1 -> DelayEnable/2
  [task_time_s] -> DelayEnable/3
  Constant2/1 -> Equal/2
  [VINP_APSStaSys_enum] -> Equal/1
  Equal/1 -> OR/1
  OR/1 -> AND1/3
  [VINP_APSVMCReqA_flg] -> AND1/1
  Constant3/1 -> Equal1/2
  Equal1/1 -> OR/2
  [VINP_APSStaSys_enum] -> Equal1/1
  [VVMC_APSCtrlAvail_flg] -> AND1/2
  AND1/1 -> VVMC_APSActive_flg/1  "VVMC_APSActive_flg"
  VINP_APSStaSys_enum/1 -> [VINP_APSStaSys_enum]
  VTQD_ExtDoorAllow_flg/1 -> [VTQD_ExtDoorAllow_flg]
  Constant4/1 -> DelayEnable2/2
  DelayEnable2/1 -> [VVMC_APSDoorCtrlAllow_flg]  "VVMC_APSDoorCtrlAllow_flg"
  [task_time_s] -> DelayEnable2/3
  [VTQD_ExtDoorAllow_flg] -> DelayEnable2/1
  [VVMC_APSDoorCtrlAllow_flg] -> AND/3

== system vmc/VMC/VMC/APS function/Signal Rounting ==
  VINP_SCPSystemMode_enum : Inport
  VVMC_APSActive_flg : Inport  Port=2
  VVMC_ADASActive_flg : Inport  Port=3
  BINP_APM_outputs : Inport  Port=4
  VTQD_GearActualPosn_enum : Inport  Port=5
  VTQD_APSStaSys_enum : Inport  Port=6
  VTQD_APSDecReqA_flg : Inport  Port=7
  VTQD_APSDecReq_mps2 : Inport  Port=8
  VTQD_APSReq_enum : Inport  Port=9
  Ground{,1..3} (4 alike) : Ground
  Signal Determination VINP_APSDecReqAtest_flg : Subsystem
  Signal Determination VINP_APSDecReqtest_mps2 : Subsystem
  Signal Determination VINP_APSReqtest_enum : Subsystem
  Signal Determination VINP_APSStaSystemtest_enum : Subsystem
  Terminator{,1..3} (4 alike) : Terminator
  VVMC_APSStaSys_enum : Outport
  VVMC_APSDecReqA_flg : Outport  Port=2
  VVMC_APSDecReq_mps2 : Outport  Port=3
  VVMC_APSReq_enum : Outport  Port=4
  wires:
  [VINP_SCPSystemMode_enum] -> Signal Determination VINP_APSDecReqtest_mps2/3(VINP_SCPSystemMode_enum)
  Signal Determination VINP_APSDecReqAtest_flg/1(SignalOutp) -> VVMC_APSDecReqA_flg/1  "VVMC_APSDecReqA_flg"
  Signal Determination VINP_APSReqtest_enum/1(SignalOutp) -> VVMC_APSReq_enum/1  "VVMC_APSReq_enum"
  [VTQD_APSDecReq_mps2] -> Signal Determination VINP_APSDecReqtest_mps2/2(SignalInput2)
  [VTQD_APSReq_enum] -> Signal Determination VINP_APSReqtest_enum/2(SignalInput2)
  Ground2/1 -> Signal Determination VINP_APSDecReqtest_mps2/1(SignalInput1)
  [VINP_SCPSystemMode_enum] -> Signal Determination VINP_APSReqtest_enum/3(VINP_SCPSystemMode_enum)
  Signal Determination VINP_APSStaSystemtest_enum/1(SignalOutp) -> VVMC_APSStaSys_enum/1  "VVMC_APSStaSys_enum"
  [VINP_SCPSystemMode_enum] -> Signal Determination VINP_APSDecReqAtest_flg/3(VINP_SCPSystemMode_enum)
  Signal Determination VINP_APSDecReqtest_mps2/1(SignalOutp) -> VVMC_APSDecReq_mps2/1  "VVMC_APSDecReq_mps2"
  VINP_SCPSystemMode_enum/1 -> [VINP_SCPSystemMode_enum]
  Ground/1 -> Signal Determination VINP_APSStaSystemtest_enum/1(SignalInput1)
  Ground1/1 -> Signal Determination VINP_APSDecReqAtest_flg/1(SignalInput1)
  Ground3/1 -> Signal Determination VINP_APSReqtest_enum/1(SignalInput1)
  VVMC_APSActive_flg/1 -> [VVMC_APSActive_flg]
  VVMC_ADASActive_flg/1 -> [VVMC_ADASActive_flg]
  [VVMC_APSActive_flg] -> Signal Determination VINP_APSStaSystemtest_enum/4(VVMC_APSActive_flg)
  [VVMC_ADASActive_flg] -> Signal Determination VINP_APSStaSystemtest_enum/5(VVMC_ADASActive_flg)
  [VTQD_APSDecReqA_flg] -> Signal Determination VINP_APSDecReqAtest_flg/2(SignalInput2)
  [VVMC_APSActive_flg] -> Signal Determination VINP_APSDecReqAtest_flg/4(VVMC_APSActive_flg)
  [VVMC_ADASActive_flg] -> Signal Determination VINP_APSDecReqAtest_flg/5(VVMC_ADASActive_flg)
  [VVMC_APSActive_flg] -> Signal Determination VINP_APSDecReqtest_mps2/4(VVMC_APSActive_flg)
  [VVMC_ADASActive_flg] -> Signal Determination VINP_APSDecReqtest_mps2/5(VVMC_ADASActive_flg)
  [VVMC_APSActive_flg] -> Signal Determination VINP_APSReqtest_enum/4(VVMC_APSActive_flg)
  [VVMC_ADASActive_flg] -> Signal Determination VINP_APSReqtest_enum/5(VVMC_ADASActive_flg)
  [VTQD_APSStaSys_enum] -> Signal Determination VINP_APSStaSystemtest_enum/2(SignalInput2)
  VTQD_GearActualPosn_enum/1 -> [VTQD_GearActualPosn_enum]
  BINP_APM_outputs/1 -> [BINP_APM_outputs]
  [VTQD_GearActualPosn_enum] -> Signal Determination VINP_APSStaSystemtest_enum/6(VTQD_GearActualPosn_enum)
  [VINP_SCPSystemMode_enum] -> Signal Determination VINP_APSStaSystemtest_enum/3(VINP_SCPSystemMode_enum)
  [BINP_APM_outputs] -> Terminator/1
  [BINP_APM_outputs] -> Terminator1/1
  [BINP_APM_outputs] -> Terminator2/1
  [BINP_APM_outputs] -> Terminator3/1
  VTQD_APSReq_enum/1 -> [VTQD_APSReq_enum]
  VTQD_APSDecReqA_flg/1 -> [VTQD_APSDecReqA_flg]
  VTQD_APSStaSys_enum/1 -> [VTQD_APSStaSys_enum]
  VTQD_APSDecReq_mps2/1 -> [VTQD_APSDecReq_mps2]

== system vmc/VMC/VMC/CruiseControlFunction/CCActiveDetermination ==
  VINP_ZoneSpdCtrlMode_enum : Inport
  VVMC_FeatArbitrFinal_enum : Inport  Port=2
  VTQD_ExternalTqAllow_flg : Inport  Port=3
  VINP_SWCSetdownSta_flg : Inport  Port=4
  VINP_SWCResUpSta_flg : Inport  Port=5
  VINP_VehSpeed_kph : Inport  Port=6
  VVMC_FeatSetSpdForCalcu_kph : Inport  Port=7
  VINP_BrakeSWGPIO_flg : Inport  Port=8
  VINP_SWCCANCELSta_flg : Inport  Port=9
  VINP_BrkSwSta_flg : Inport  Port=10
  VINP_ADASAEBSta_enum : Inport  Port=11
  VVMC_CCPedalOvrd_flg : Inport  Port=12
  VTQD_GearActualPosn_enum : Inport  Port=13
  AND : Logic  AllPortsSameDT=off  OutDataTypeStr=boolean
  Cast To Single : DataTypeConversion  OutDataTypeStr=uint8
  Cast To Single1 : DataTypeConversion  OutDataTypeStr=boolean
  Cast To Single2 : DataTypeConversion  OutDataTypeStr=boolean
  Chart : Stateflow chart  TreatAsAtomicUnit=on
  Constant : Constant  Value=KVMC_CCActiveMetSpdHi_kph
  Constant1 : Constant  Value=KVMC_CCActiveMetSpdLo_kph
  Constant2 : Constant  Value=KVMC_CCMSASpdWar_kph
  Constant3 : Constant  Value=ENUM_FEATARBITRSTA_CC
  Constant4 : Constant  Value=TRUE
  Constant5 : Constant  Value=FALSE
  Constant6 : Constant  Value=ENUM_CCCRLSTA_ACTIVE
  Constant7 : Constant  Value=ENUM_ADASAEBSTA_ACTIVE
  Constant8 : Constant  Value=ENUM_GEARACTUALPOSN_D
  Constant9 : Constant  Value=ZERO_FLOAT
  Delay : Delay  DelayLength=1
  Detect Decrease : simulink/Logic and Bit Operations/Detect Decrease  vinit=0.0  OutDataTypeStr=boolean
  Detect Decrease1 : simulink/Logic and Bit Operations/Detect Decrease  vinit=0.0  OutDataTypeStr=boolean
  Detect Decrease2 : simulink/Logic and Bit Operations/Detect Decrease  vinit=0.0  OutDataTypeStr=boolean
  Relational Operator : RelationalOperator  Operator===  OutDataTypeStr=boolean  RndMeth=Simplest
  Relational Operator1 : RelationalOperator  Operator===  OutDataTypeStr=boolean  RndMeth=Simplest
  u2 > 0 : Switch  Criteria=u2 > Threshold
  VVMC_CCCtrlSta_enum : Outport
  VVMC_CCSpdWar_flg : Outport  Port=2
  VVMC_CruzActive_flg : Outport  Port=3
  wires:
  Delay/1 -> Chart/16(VVMC_CCPedalOvrd_flg)
  [VVMC_CCPedalOvrd_flg] -> Delay/1
  VVMC_CCPedalOvrd_flg/1 -> [VVMC_CCPedalOvrd_flg]
  Constant7/1 -> Chart/14(ENUM_ADASAEBSTA_ACTIVE)
  [VINP_ADASAEBSta_enum] -> Chart/13(VINP_ADASAEBSta_enum)
  VINP_ADASAEBSta_enum/1 -> [VINP_ADASAEBSta_enum]
  Relational Operator1/1 -> AND/2
  Relational Operator/1 -> AND/1
  [VVMC_CCCtrlSta_enum] -> Relational Operator1/1
  Constant6/1 -> Relational Operator1/2
  Constant5/1 -> u2 > 0/3
  Constant4/1 -> u2 > 0/1
  AND/1 -> u2 > 0/2
  [VINP_ZoneSpdCtrlMode_enum] -> Chart/1(VINP_ZoneSpdCtrlMode_enum)
  VINP_ZoneSpdCtrlMode_enum/1 -> [VINP_ZoneSpdCtrlMode_enum]
  Constant3/1 -> Relational Operator/2
  Constant/1 -> Chart/4(KVMC_CCActiveMetSpdHi_kph)
  [VINP_VehSpeed_kph] -> Chart/5(VINP_VehSpeed_kph)
  Constant1/1 -> Chart/6(KVMC_CCActiveMetSpdLo_kph)
  [VINP_SWCSetdownSta_flg] -> Detect Decrease/1
  [VVMC_FeatSetSpdForCalcu_kph] -> Chart/7(VVMC_FeatSetSpdForCalcu_kph)
  Constant2/1 -> Chart/8(KVMC_CCMSASpdWar_kph)
  [VTQD_ExternalTqAllow_flg] -> Chart/2(VTQD_ExternalTqAllow_flg)
  [VVMC_FeatArbitrFinal_enum] -> Relational Operator/1
  [VINP_BrakeSWGPIO_flg] -> Chart/9(VINP_BrakeSWGPIO_flg)
  [VINP_SWCCANCELSta_flg] -> Detect Decrease1/1
  [VINP_SWCResUpSta_flg] -> Detect Decrease2/1
  Chart/1(VVMC_CCCtrlSta_enum) -> Cast To Single/1
  Chart/2(VVMC_CCSpdWar_flg) -> Cast To Single1/1
  u2 > 0/1 -> Cast To Single2/1
  VVMC_FeatArbitrFinal_enum/1 -> [VVMC_FeatArbitrFinal_enum]
  VTQD_ExternalTqAllow_flg/1 -> [VTQD_ExternalTqAllow_flg]
  VINP_SWCSetdownSta_flg/1 -> [VINP_SWCSetdownSta_flg]
  VINP_SWCResUpSta_flg/1 -> [VINP_SWCResUpSta_flg]
  VINP_VehSpeed_kph/1 -> [VINP_VehSpeed_kph]
  VVMC_FeatSetSpdForCalcu_kph/1 -> [VVMC_FeatSetSpdForCalcu_kph]
  VINP_BrakeSWGPIO_flg/1 -> [VINP_BrakeSWGPIO_flg]
  VINP_SWCCANCELSta_flg/1 -> [VINP_SWCCANCELSta_flg]
  VINP_BrkSwSta_flg/1 -> [VINP_BrkSwSta_flg]
  [VVMC_CCCtrlSta_enum] -> VVMC_CCCtrlSta_enum/1
  [VVMC_CCSpdWar_flg] -> VVMC_CCSpdWar_flg/1
  [VVMC_CruzActive_flg] -> VVMC_CruzActive_flg/1
  Detect Decrease/1 -> Chart/3(VVMC_DetectSWCSetDown_flg)  "VVMC_DetectSWCSetDown_flg"
  Detect Decrease1/1 -> Chart/10(VVMC_DetectSWCCANCEL_flg)  "VVMC_DetectSWCCANCEL_flg"
  Detect Decrease2/1 -> Chart/12(VVMC_DetectSWCResUp_flg)  "VVMC_DetectSWCResUp_flg"
  Cast To Single1/1 -> [VVMC_CCSpdWar_flg]  "VVMC_CCSpdWar_flg"
  Cast To Single2/1 -> [VVMC_CruzActive_flg]  "VVMC_CruzActive_flg"
  Cast To Single/1 -> [VVMC_CCCtrlSta_enum]  "VVMC_CCCtrlSta_enum"
  [VINP_BrkSwSta_flg] -> Chart/11(VINP_BrkSwSta_flg)
  VTQD_GearActualPosn_enum/1 -> [VTQD_GearActualPosn_enum]
  [VTQD_GearActualPosn_enum] -> Chart/17(VTQD_GearActualPosn_enum)
  Constant8/1 -> Chart/18(ENUM_GEARACTUALPOSN_D)
  Constant9/1 -> Chart/15(ZERO_FLOAT)

== system vmc/VMC/VMC/CruiseControlFunction/CCDemandTorqueCalculation ==
  VVMC_FeatSetSpdForCalcu_kph : Inport
  VINP_VehSpeed_kph : Inport  Port=2
  VVMC_CruzActive_flg : Inport  Port=3
  VTQD_DriverWhlTqDem_Nm : Inport  Port=4
  VVMC_LongAcc_Gps : Inport  Port=5
  VVMC_CCPedalOvrd_flg : Inport  Port=6
  VVMC_CalMeterSpeed_kph : Inport  Port=7
  VVMC_FeatArbitrFinal_enum : Inport  Port=8
  VVMC_ActACCRequiredAccel_mps2 : Inport  Port=9
  VVMC_MeterIndSpeedForCalcu_kph : Inport  Port=10
  VVMC_SafetyCtrl_flg : Inport  Port=11
  VTQR_FrTMTqReq_Nm : Inport  Port=12
  VTQR_RrTMTqReq_Nm : Inport  Port=13
  VVMC_TotalAvailBrkRgnTq_Nm : Inport  Port=14
  AND12 : Logic  AllPortsSameDT=off  OutDataTypeStr=boolean
  Abs3 : Abs
  Abs4 : Abs
  Add{8,12,16,20..21} (5 alike) : Sum
  Add22 : Sum  Inputs=+-
  Add23 : Sum  Inputs=+-
  Cast To Single4 : DataTypeConversion  OutDataTypeStr=single
  Cast To Single5 : DataTypeConversion  OutDataTypeStr=single
  Constant1 : Constant  Value=KVMC_CCTqUpLim_Nm
  Constant104 : Constant  Value=ZERO_FLOAT
  Constant105 : Constant  Value=KTQD_RrTMTotalGearRatio_gain
  Constant106 : Constant  Value=KTQR_RrTMGearEff_c
  Constant107 : Constant  Value=KVMC_GravityValue_mps2
  Constant2 : Constant  Value=KVMC_CCTqLowLim_Nm
  Constant3 : Constant  Value=ZERO_FLOAT
  Constant36 : Constant  Value=KVMC_AccDevLowLim_mps2
  Constant38 : Constant  Value=KVMC_AccDevUpLim_mps2
  Constant4 : Constant  Value=KVMC_CCDISCPGainSW_flg
  Constant40 : Constant  Value=KVMC_CCSpdDevUpLim_kph
  Constant5 : Constant  Value=KVMC_CCTqUpLim_Nm
  Constant56 : Constant  Value=KVMC_CCSpdDevLowLim_kph
  Constant58 : Constant  Value=KVMC_Veh2MeterSpdFactor_enum
  Constant59 : Constant  Value=KVMC_Veh2MeterSpdOffset_enum
  Constant6 : Constant  Value=KVMC_CCTqLowLim_Nm
  Constant64 : Constant  Value=KVMC_TqSafetyCtrl_flg
  Constant65 : Constant  Value=KVMC_Veh2MeterSpdLoFactor_enum
  Constant7 : Constant  Value=ZERO_FLOAT
  Constant71 : Constant  Value=KTQR_FrTMGearEff_c
  Constant76 : Constant  Value=KTQD_FrTMTotalGearRatio_gain
  Data Type Conversion1 : DataTypeConversion  OutDataTypeStr=single
  Detect Decrease3 : simulink/Logic and Bit Operations/Detect Decrease  vinit=0.0  OutDataTypeStr=boolean
  Detect Increase3 : simulink/Logic and Bit Operations/Detect Increase  vinit=0.0  OutDataTypeStr=boolean
  Divide11 : Product  Inputs=**
  Divide12 : Product  Inputs=**
  Divide4 : Product  Inputs=***
  Divide7 : Product  Inputs=***
  InitialCondition: 1 : UnitDelay  SampleTime=-1  HasFrameUpgradeWarning=on
  Logical Operator1 : Logic  Operator=OR  AllPortsSameDT=off  OutDataTypeStr=boolean
  MVMC_DISCDeltaTqIGain_Z_Nm : Lookup_n-D  BreakpointsForDimension1=AVMC_DISCDeltaTqIGain_Y_mps2  BreakpointsForDimension2=AVMC_DISCDeltaTqIGain_X_kph  Table=MVMC_DISCDeltaTqIGain_Z_Nm  InternalRulePriority=Speed  RndMeth=Simplest  InputSameDT=on
      settings: InputPortMap=u0,u1
  MVMC_DISCDeltaTqPGain_Z_Nm : Lookup_n-D  BreakpointsForDimension1=AVMC_DISCDeltaTqPGain_Y_kph  BreakpointsForDimension2=AVMC_DISCDeltaTqPGain_X_kph  BreakpointsForDimension3=[5, 7]  Table=MVMC_DISCDeltaTqPGain_Z_Nm  ExtrapMethod=Clip  InternalRulePriority=Speed  RndMeth=Simplest  InputSameDT=on
      settings: InputPortMap=u0,u1
  Max : MinMax  Function=max  Inputs=2
  Max1 : MinMax  Function=max  Inputs=2
  Product2 : Product
  Relational Operator18 : RelationalOperator  Operator=<=  OutDataTypeStr=boolean  RndMeth=Simplest
  Saturation Dynamic{1,7..9} (4 alike) : simulink/Discontinuities/Saturation Dynamic  OutMin=[]  OutMax=[]  OutDataTypeStr=Inherit: Same as second input  OutDataType=fixdt(1, 16)  OutScaling=2^-10  DoSatur=off
  Switch{,2,5,7} (4 alike) : Switch  Criteria=u2 > Threshold
  Switch1 : Switch  Criteria=u2 > Threshold  Threshold=KVMC_Veh2MeterSpdLoBdy_kph
  Unit Delay3 : UnitDelay  SampleTime=-1  HasFrameUpgradeWarning=on
  u2 > 0 (3)1 : Switch  Criteria=u2 > Threshold
  u2 > 0 (4)1 : Switch  Criteria=u2 > Threshold
  VVMC_CruzWhlTqCal_Nm : Outport
  wires:
  VVMC_FeatSetSpdForCalcu_kph/1 -> [VVMC_FeatSetSpdForCalcu_kph]
  VTQD_DriverWhlTqDem_Nm/1 -> [VTQD_DriverWhlTqDem_Nm]
  VVMC_CruzActive_flg/1 -> [VVMC_CruzActive_flg]
  VINP_VehSpeed_kph/1 -> [VINP_VehSpeed_kph]
  [VVMC_CruzWhlTqCal_Nm] -> VVMC_CruzWhlTqCal_Nm/1
  VVMC_LongAcc_Gps/1 -> [VVMC_LongAcc_Gps]
  VVMC_CCPedalOvrd_flg/1 -> [VVMC_CCPedalOvrd_flg]
  VVMC_CalMeterSpeed_kph/1 -> [VVMC_CalMeterSpeed_kph]
  VVMC_FeatArbitrFinal_enum/1 -> [VVMC_FeatArbitrFinal_enum]
  VVMC_ActACCRequiredAccel_mps2/1 -> [VVMC_CCReqAcc_mps2]
  VVMC_MeterIndSpeedForCalcu_kph/1 -> [VVMC_MeterIndSpeedForCalcu_kph]
  VVMC_SafetyCtrl_flg/1 -> [VVMC_SafetyCtrl_flg]
  Switch5/1 -> Cast To Single5/1
  Detect Decrease3/1 -> Logical Operator1/2
  Divide4/1 -> Add16/1
  [VVMC_CruzActive_flg] -> Detect Increase3/1
  [VVMC_FeatSetSpdForCalcu_kph] -> MVMC_DISCDeltaTqPGain_Z_Nm/2
  Data Type Conversion1/1 -> Add23/1
  u2 > 0 (3)1/1 -> Switch5/1
  Constant71/1 -> Divide4/3
  Constant106/1 -> Divide7/3
  [VVMC_SafetyCtrl_flg] -> AND12/2
  Saturation Dynamic9/1 -> MVMC_DISCDeltaTqPGain_Z_Nm/1
  Relational Operator18/1 -> u2 > 0 (4)1/2
  [VVMC_LastCCWhlTqCalW_Nm] -> Abs3/1, u2 > 0 (4)1/1
  u2 > 0 (4)1/1 -> u2 > 0 (3)1/1
  [VTQR_RrTMTqReq_Nm] -> Divide7/1
  [VVMC_LastCCWhlTqCalW_Nm] -> Add12/1
  MVMC_DISCDeltaTqIGain_Z_Nm/1 -> [VVMC_CCIGainDeltaTq_Nm]
  Add23/1 -> Saturation Dynamic9/2
  Constant104/1 -> Switch5/3
  InitialCondition: 1/1 -> [VVMC_LastCCWhlTqCalW_Nm]  "VVMC_LastCruzWhlTqCal_Nm"
  Detect Increase3/1 -> Logical Operator1/1
  [VINP_VehSpeed_kph] -> MVMC_DISCDeltaTqIGain_Z_Nm/2
  [VVMC_CCIGainDeltaTq_Nm] -> Add12/2
  Abs4/1 -> Relational Operator18/2
  Saturation Dynamic7/1 -> InitialCondition: 1/1, Add21/2
  Abs3/1 -> Relational Operator18/1
  [VTQR_FrTMTqReq_Nm] -> Divide4/1
  Saturation Dynamic8/1 -> MVMC_DISCDeltaTqIGain_Z_Nm/1
  [VVMC_CCIGainDeltaTq_Nm] -> Add20/2
  Constant76/1 -> Divide4/2
  Divide7/1 -> Add16/2
  AND12/1 -> u2 > 0 (3)1/2
  Add20/1 -> Switch7/1
  Constant105/1 -> Divide7/2
  [VVMC_CruzActive_flg] -> Switch5/2
  [VVMC_CCPedalOvrd_flg] -> Unit Delay3/1
  Cast To Single5/1 -> Saturation Dynamic7/2
  Switch7/1 -> Cast To Single4/1
  Add12/1 -> Switch7/3
  Constant40/1 -> Saturation Dynamic9/1
  Constant5/1 -> Saturation Dynamic7/1
  Add16/1 -> Add20/1
  Unit Delay3/1 -> Detect Decrease3/1
  [VVMC_CCReqAcc_mps2] -> Add22/1
  Add22/1 -> Saturation Dynamic8/2
  Constant107/1 -> Product2/2
  Constant64/1 -> AND12/1
  [VVMC_FeatSetSpdForCalcu_kph] -> Data Type Conversion1/1
  Logical Operator1/1 -> Switch7/2
  Constant38/1 -> Saturation Dynamic8/1
  Product2/1 -> Add22/2
  [VVMC_LongAcc_Gps] -> Product2/1
  Constant36/1 -> Saturation Dynamic8/3
  Constant6/1 -> Max/1
  Constant56/1 -> Saturation Dynamic9/3
  Cast To Single4/1 -> u2 > 0 (4)1/3, Abs4/1, u2 > 0 (3)1/3
  VTQR_FrTMTqReq_Nm/1 -> [VTQR_FrTMTqReq_Nm]
  VTQR_RrTMTqReq_Nm/1 -> [VTQR_RrTMTqReq_Nm]
  VVMC_TotalAvailBrkRgnTq_Nm/1 -> [VVMC_TotalAvailBrkRgnTq_Nm]
  [VVMC_TotalAvailBrkRgnTq_Nm] -> Max/2
  Max/1 -> Saturation Dynamic7/3
  Switch/1 -> [VVMC_CCPGainDeltaTq_Nm]
  Switch2/1 -> Add21/1
  [VVMC_CCPGainDeltaTq_Nm] -> Switch2/1
  Constant4/1 -> Switch2/2
  Constant7/1 -> Switch2/3
  Saturation Dynamic1/1 -> [VVMC_CruzWhlTqCal_Nm]  "VVMC_CruzWhlTqCal_Nm"
  [VINP_VehSpeed_kph] -> Divide11/2, Switch1/2, Divide12/1
  Switch1/1 -> Add23/2
  Constant59/1 -> Add8/1
  Add8/1 -> Switch1/1
  Constant58/1 -> Divide11/1
  Constant65/1 -> Divide12/2
  Divide11/1 -> Add8/2
  Divide12/1 -> Switch1/3
  Max1/1 -> Saturation Dynamic1/3
  [VVMC_TotalAvailBrkRgnTq_Nm] -> Max1/2
  Constant2/1 -> Max1/1
  Constant1/1 -> Saturation Dynamic1/1
  Add21/1 -> Saturation Dynamic1/2
  [VVMC_CruzActive_flg] -> Switch/2
  MVMC_DISCDeltaTqPGain_Z_Nm/1 -> Switch/1
  Constant3/1 -> Switch/3

== system vmc/VMC/VMC/CruiseControlFunction/CCTorqueSourceDetermination ==
  VTQD_DriverWhlTqDem_Nm : Inport
  VVMC_CruzWhlTqCal_Nm : Inport  Port=2
  VTQD_LowIdleAccPedal_flg : Inport  Port=3
  VINP_RegenMode_enum : Inport  Port=4
  VVMC_FeatArbitrFinal_enum : Inport  Port=5
  task_time_s : Inport  Port=6
  AND1 : Logic  Inputs=3  AllPortsSameDT=off  OutDataTypeStr=boolean
  Add : Sum
  Constant20 : Constant  Value=FALSE
  Constant21 : Constant  Value=ENUM_FEATARBITRSTA_CC
  Constant22 : Constant  Value=TRUE
  Constant23 : Constant  Value=KVMC_ACCPedalOvrdRestTime_s
  DelayEnable : hcu_lib/Basic_Blocks/DelayEnable
  Direct Lookup Table (n-D)1 : LookupNDDirect  NumberOfTableDimensions=1  Table=MVMC_ACCPedalOvrdTqHys_Y_Nm
  NOT2 : Logic  Operator=NOT  AllPortsSameDT=off  OutDataTypeStr=boolean
  OR1 : Logic  Operator=OR  AllPortsSameDT=off  OutDataTypeStr=boolean
  Relational Operator6 : RelationalOperator  Operator===  OutDataTypeStr=boolean  RndMeth=Simplest
  Relational Operator7 : RelationalOperator  Operator=>  OutDataTypeStr=boolean  RndMeth=Simplest
  Relational Operator8 : RelationalOperator  Operator=<=  OutDataTypeStr=boolean  RndMeth=Simplest
  SR_Latch : hcu_lib/Basic_Blocks/SR_Latch
  u2 > 0 (1) : Switch  Criteria=u2 > Threshold
  u2 > 0 (2) : Switch  Criteria=u2 > Threshold
  VVMC_CruzWhlTqReq_Nm : Outport
  VVMC_CCPedalOvrd_flg : Outport  Port=2
  wires:
  VTQD_DriverWhlTqDem_Nm/1 -> [VTQD_DriverWhlTqDem_Nm]
  VVMC_CruzWhlTqCal_Nm/1 -> [VVMC_CruzWhlTqCal_Nm]
  [VVMC_CruzWhlTqReq_Nm] -> VVMC_CruzWhlTqReq_Nm/1
  VTQD_LowIdleAccPedal_flg/1 -> [VTQD_LowIdleAccPedal_flg]
  [VVMC_CCPedalOvrd_flg] -> VVMC_CCPedalOvrd_flg/1
  [task_time_s] -> DelayEnable/3
  [VTQD_LowIdleAccPedal_flg] -> NOT2/1
  [VTQD_DriverWhlTqDem_Nm] -> u2 > 0 (1)/1
  [VVMC_CruzWhlTqCal_Nm] -> u2 > 0 (1)/3
  [VVMC_CruzWhlTqCal_Nm] -> Relational Operator8/2
  [VVMC_CruzWhlTqCal_Nm] -> Add/1
  u2 > 0 (2)/1 -> [VVMC_CCPedalOvrd_flg]
  Add/1 -> Relational Operator7/2
  [VTQD_DriverWhlTqDem_Nm] -> Relational Operator7/1
  [VVMC_FeatArbitrFinal_enum] -> Relational Operator6/1
  OR1/1 -> SR_Latch/2
  Relational Operator8/1 -> DelayEnable/1
  Constant23/1 -> DelayEnable/2
  u2 > 0 (1)/1 -> [VVMC_CruzWhlTqReq_Nm]
  Relational Operator7/1 -> SR_Latch/1
  [VVMC_CCPedalTqEnOvrd_flg] -> AND1/3
  NOT2/1 -> AND1/2
  Constant20/1 -> u2 > 0 (2)/3
  Relational Operator6/1 -> AND1/1
  [VINP_RegenMode_enum] -> Direct Lookup Table (n-D)1/1
  [VTQD_DriverWhlTqDem_Nm] -> Relational Operator8/1
  DelayEnable/1 -> OR1/1
  SR_Latch/1 -> [VVMC_CCPedalTqEnOvrd_flg]
  [VTQD_LowIdleAccPedal_flg] -> OR1/2
  AND1/1 -> u2 > 0 (1)/2, u2 > 0 (2)/2
  Constant21/1 -> Relational Operator6/2
  Direct Lookup Table (n-D)1/1 -> Add/2
  Constant22/1 -> u2 > 0 (2)/1
  VINP_RegenMode_enum/1 -> [VINP_RegenMode_enum]
  VVMC_FeatArbitrFinal_enum/1 -> [VVMC_FeatArbitrFinal_enum]
  task_time_s/1 -> [task_time_s]

== system vmc/VMC/VMC/IMU/IMU memorized offset result ==
  VINP_MemOffsetGyroX_raw16 : Inport
  VINP_MemOffsetGyroY_raw16 : Inport  Port=2
  VINP_MemOffsetGyroZ_raw16 : Inport  Port=3
  VINP_MemOffsetAccX_raw16 : Inport  Port=4
  VINP_MemOffsetAccY_raw16 : Inport  Port=5
  VINP_MemOffsetAccZ_raw16 : Inport  Port=6
  ACCEL_FS_SEL = 001 SENSITIVITY = 2000 LSB/g : Constant  Value=2000
  Constant6 : Constant  Value=ONE_FLOAT  OutDataTypeStr=single
  Data Type Conversion : DataTypeConversion  OutDataTypeStr=uint16
  Data Type Conversion{1..6} (6 alike) : DataTypeConversion  OutDataTypeStr=single
  Data Type Conversion7 : DataTypeConversion  OutDataTypeStr=uint16
  Divide{,1..5} (6 alike) : Product  Inputs=**
  GYRO_FS_SEL = 0001 SENSITIVITY = 50 LSB/dps : Constant  Value=50
  Math Function{,1..5} (6 alike) : Math  Operator=reciprocal  SaturateOnIntegerOverflow=on
  Plus : Sum  Inputs=+-
  VVMC_MemOffsetGyroX_Dps : Outport
  VVMC_MemOffsetGyroY_Dps : Outport  Port=2
  VVMC_MemOffsetGyroZ_Dps : Outport  Port=3
  VVMC_MemOffsetAccX_G : Outport  Port=4
  VVMC_MemOffsetAccY_G : Outport  Port=5
  VVMC_MemOffsetAccZ_G : Outport  Port=6
  wires:
  VINP_MemOffsetGyroX_raw16/1 -> [VINP_MemOffsetGyroX_raw16]
  VINP_MemOffsetGyroY_raw16/1 -> [VINP_MemOffsetGyroY_raw16]
  [VINP_MemOffsetGyroX_raw16] -> Divide/1
  [VVMC_GyroFSCalSet_enum] -> Data Type Conversion1/1
  GYRO_FS_SEL = 0001 SENSITIVITY = 50 LSB/dps/1 -> Data Type Conversion/1
  Data Type Conversion/1 -> [VVMC_GyroFSCalSet_enum]  "VVMC_GyroFSCalSet_enum"
  [VVMC_GyroFSCalSet_enum] -> Data Type Conversion2/1
  [VINP_MemOffsetGyroY_raw16] -> Divide1/1
  [VINP_MemOffsetGyroZ_raw16] -> Divide2/1
  [VVMC_GyroFSCalSet_enum] -> Data Type Conversion3/1
  [VVMC_AccFSCalSet_enum] -> Data Type Conversion4/1
  [VINP_MemOffsetAccX_raw16] -> Divide3/1
  [VINP_MemOffsetAccY_raw16] -> Divide4/1
  [VVMC_AccFSCalSet_enum] -> Data Type Conversion5/1
  [VVMC_AccFSCalSet_enum] -> Data Type Conversion6/1
  [VINP_MemOffsetAccZ_raw16] -> Divide5/1
  Data Type Conversion7/1 -> [VVMC_AccFSCalSet_enum]  "VVMC_AccFSCalSet_enum"
  ACCEL_FS_SEL = 001 SENSITIVITY = 2000 LSB/g/1 -> Data Type Conversion7/1
  Divide/1 -> [VVMC_MemOffsetGyroX_Dps]  "VVMC_MemOffsetGyroX_Dps"
  Divide1/1 -> [VVMC_MemOffsetGyroY_Dps]  "VVMC_MemOffsetGyroY_Dps"
  Divide2/1 -> [VVMC_MemOffsetGyroZ_Dps]  "VVMC_MemOffsetGyroZ_Dps"
  Divide3/1 -> [VVMC_MemOffsetAccX_G]  "VVMC_MemOffsetAccX_G"
  Plus/1 -> [VVMC_MemOffsetAccZ_G]  "VVMC_MemOffsetAccZ_G"
  Divide5/1 -> Plus/1
  Constant6/1 -> Plus/2
  [VVMC_MemOffsetGyroX_Dps] -> VVMC_MemOffsetGyroX_Dps/1
  [VVMC_MemOffsetGyroY_Dps] -> VVMC_MemOffsetGyroY_Dps/1
  [VVMC_MemOffsetGyroZ_Dps] -> VVMC_MemOffsetGyroZ_Dps/1
  [VVMC_MemOffsetAccX_G] -> VVMC_MemOffsetAccX_G/1
  [VVMC_MemOffsetAccY_G] -> VVMC_MemOffsetAccY_G/1
  [VVMC_MemOffsetAccZ_G] -> VVMC_MemOffsetAccZ_G/1
  Divide4/1 -> [VVMC_MemOffsetAccY_G]  "VVMC_MemOffsetAccY_G"
  VINP_MemOffsetGyroZ_raw16/1 -> [VINP_MemOffsetGyroZ_raw16]
  VINP_MemOffsetAccX_raw16/1 -> [VINP_MemOffsetAccX_raw16]
  VINP_MemOffsetAccY_raw16/1 -> [VINP_MemOffsetAccY_raw16]
  VINP_MemOffsetAccZ_raw16/1 -> [VINP_MemOffsetAccZ_raw16]
  Math Function/1 -> Divide/2
  Math Function1/1 -> Divide1/2
  Math Function2/1 -> Divide2/2
  Math Function3/1 -> Divide3/2
  Math Function4/1 -> Divide4/2
  Math Function5/1 -> Divide5/2
  Data Type Conversion1/1 -> Math Function/1
  Data Type Conversion2/1 -> Math Function1/1
  Data Type Conversion3/1 -> Math Function2/1
  Data Type Conversion4/1 -> Math Function3/1
  Data Type Conversion5/1 -> Math Function4/1
  Data Type Conversion6/1 -> Math Function5/1
